simulink model "pid3_2"  (R2023b)
settings: Solver=VariableStepAuto  StartTime=0.0  StopTime=150  RelTol=1e-3
libraries: simulink x2
settings Model: Creator=21917  LastModifiedBy=21917

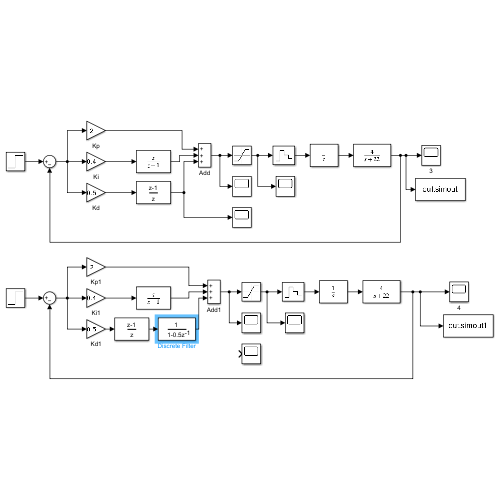
[thumbnail: Simulink's stored preview of the top-level diagram]
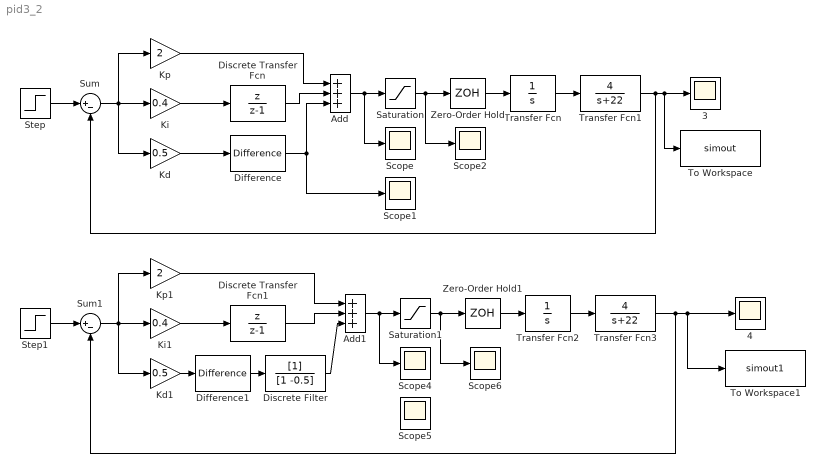
== system pid3_2 ==
  3 : Scope
  4 : Scope
  Add : Sum  Inputs=+++
  Add1 : Sum  Inputs=+++
  Difference : simulink/Discrete/Difference  ICPrevInput=0.0  OutMin=[]  OutMax=[]  OutDataType=fixdt(1, 16)  OutScaling=2^-10  DoSatur=off
  Difference1 : simulink/Discrete/Difference  ICPrevInput=0.0  OutMin=[]  OutMax=[]  OutDataType=fixdt(1, 16)  OutScaling=2^-10  DoSatur=off
  Discrete Transfer Fcn : DiscreteTransferFcn  Numerator=[1 0]  Denominator=[1 -1]
  Discrete Transfer Fcn1 : DiscreteTransferFcn  Numerator=[1 0]  Denominator=[1 -1]
  Discrete Filter : DiscreteFilter  Denominator=[1 -0.5]
  Kd : Gain  Gain=0.5
  Kd1 : Gain  Gain=0.5
  Ki : Gain  Gain=0.4
  Ki1 : Gain  Gain=0.4
  Kp : Gain  Gain=2
  Kp1 : Gain  Gain=2
  Saturation : Saturate
  Saturation1 : Saturate
  Scope{,1..2,4..6} (6 alike) : Scope
  Step : Step  SampleTime=0
  Step1 : Step  SampleTime=0
  Sum : Sum  Inputs=|+-
  Sum1 : Sum  Inputs=|+-
  To Workspace : ToWorkspace  VariableName=simout  SaveFormat=Timeseries  SampleTime=-1
  To Workspace1 : ToWorkspace  VariableName=simout1  SaveFormat=Timeseries  SampleTime=-1
  Transfer Fcn : TransferFcn  Denominator=[1 0]
  Transfer Fcn1 : TransferFcn  Numerator=[4]  Denominator=[1 22]
  Transfer Fcn2 : TransferFcn  Denominator=[1 0]
  Transfer Fcn3 : TransferFcn  Numerator=[4]  Denominator=[1 22]
  Zero-Order Hold : ZeroOrderHold  SampleTime=-1
  Zero-Order Hold1 : ZeroOrderHold  SampleTime=-1
  wires:
  Step/1 -> Sum/1
  Sum/1 -> Kd/1, Ki/1, Kp/1
  Difference/1 -> Add/3, Scope1/1
  Kd/1 -> Difference/1
  Ki/1 -> Discrete Transfer Fcn/1
  Kp/1 -> Add/1
  Discrete Transfer Fcn/1 -> Add/2
  Add/1 -> Scope/1, Saturation/1
  Saturation/1 -> Scope2/1, Zero-Order Hold/1
  Transfer Fcn/1 -> Transfer Fcn1/1
  Zero-Order Hold/1 -> Transfer Fcn/1
  Transfer Fcn1/1 -> Sum/2, To Workspace/1, 3/1
  Transfer Fcn3/1 -> Sum1/2, To Workspace1/1, 4/1
  Transfer Fcn2/1 -> Transfer Fcn3/1
  Saturation1/1 -> Scope6/1, Zero-Order Hold1/1
  Kd1/1 -> Difference1/1
  Ki1/1 -> Discrete Transfer Fcn1/1
  Sum1/1 -> Kd1/1, Ki1/1, Kp1/1
  Discrete Transfer Fcn1/1 -> Add1/2
  Zero-Order Hold1/1 -> Transfer Fcn2/1
  Step1/1 -> Sum1/1
  Add1/1 -> Scope4/1, Saturation1/1
  Kp1/1 -> Add1/1
  Difference1/1 -> Discrete Filter/1
  Discrete Filter/1 -> Add1/3
